simulink model "testcode"  (R2013b)
settings: Solver=FixedStepDiscrete  StartTime=0.0  StopTime=0.149  FixedStep=Te  RelTol=1e-3
values from neighbouring files (symbols this model uses):
  ka = 0.1    [script.m]
  Te = 1e-3    (= 0.001)    [script.m]
settings Model: TunableVars=Te,ka  TunableVarsStorageClass=Auto,Auto  TunableVarsTypeQualifier=,  Creator=gemsdev  LastModifiedBy=gemsdev
settings DataIOCC: LoadExternalInput=on  SignalLoggingSaveFormat=ModelDataLogs
settings OptimizationCC: InlineParams=on  OptimizeModelRefInitCode=on  LifeSpan=1
settings RTWCC: SystemTargetFile=ert.tlc  TemplateMakefile=RTW.MSVCBuild  Description=Create Visual C/C++ Solution File for Embedded Coder  ProcessScript=ert_make_rtw_hook  TargetLang=C++
settings CodeAppCC: IgnoreCustomStorageClasses=off
settings ERTTargetCC: CodeReplacementLibrary=ANSI_C  GenerateSampleERTMain=on  InlinedParameterPlacement=NonHierarchical  ERTCustomFileTemplate=example_file_process.tlc

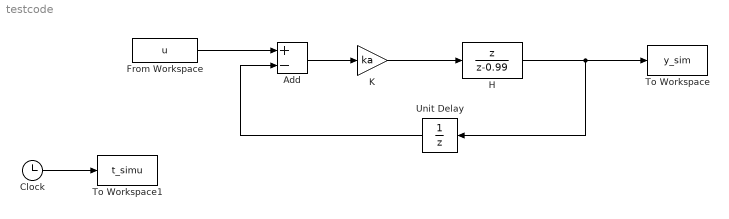
== system testcode ==
  Add : Sum  Inputs=+-  SampleTime=Te
  Clock : Clock
  From Workspace : FromWorkspace  VariableName=u  SampleTime=0
  H : DiscreteTransferFcn  Numerator=[1 0]  Denominator=[1 -0.99]  SampleTime=Te
  K : Gain  Gain=ka  SampleTime=Te
  To Workspace : ToWorkspace  VariableName=y_sim  SampleTime=-1
  To Workspace1 : ToWorkspace  VariableName=t_simu  SampleTime=-1
  Unit Delay : UnitDelay  SampleTime=Te
  wires:
  From Workspace/1 -> Add/1
  H/1 -> To Workspace/1, Unit Delay/1
  Unit Delay/1 -> Add/2
  Add/1 -> K/1
  K/1 -> H/1
  Clock/1 -> To Workspace1/1
